simulink model "log_shift_final"  (R2017b)
settings: Solver=FixedStepDiscrete  StartTime=0.0  StopTime=5  RelTol=1e-3
InitFcn:
  | load speech_signal;
  | Fs = 8000;
  | Ts = 1/Fs;
  | 
  | Data_size = 2048;
  | Address_size = log2(Data_size);
  | 
  | FFT_size = 1024
  | FFT_size_half = FFT_size;
  | Frame_shift = 256;
  | Frame_shift_bits = log2(Frame_shift);
  | 
  | Upscale = 32;
libraries: hdlsllib x16, simulink x5, dspxfrm3 x2, dspsigops x1
settings Model: Creator=Ross_admin  LastModifiedBy=s15z586
settings OptimizationCC: BlockReduction=off  ConditionallyExecuteInputs=off  DefaultParameterBehavior=Inlined
settings DebuggingCC: AlgebraicLoopMsg=error  SingleTaskRateTransMsg=error
settings HardwareCC: ProdBitPerPointer=32  ProdBitPerSizeT=32  ProdBitPerPtrDiffT=32  ProdLargestAtomicFloat=None  ProdIntDivRoundTo=Undefined  ProdEndianess=Unspecified  ProdWordSize=32  ProdHWDeviceType=ASIC/FPGA->ASIC/FPGA  TargetBitPerPointer=64  TargetBitPerSizeT=64  TargetBitPerPtrDiffT=64  TargetLongLongMode=on  TargetIntDivRoundTo=Zero  TargetEndianess=LittleEndian  TargetWordSize=64  TargetHWDeviceType=Custom Processor->MATLAB Host Computer  ProdEqTarget=off
settings CodeAppCC: StateflowObjectComments=on

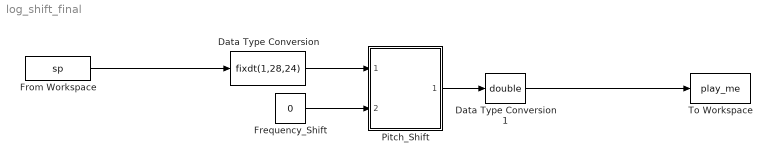
== system log_shift_final ==
  Data Type Conversion : DataTypeConversion  OutDataTypeStr=fixdt(1,28,24)
  Data Type Conversion1 : DataTypeConversion  OutDataTypeStr=double
  Frequency_Shift : Constant  Value=0  OutDataTypeStr=int16  SampleTime=Ts
  From Workspace : FromWorkspace  VariableName=sp  SampleTime=Ts
  Pitch_Shift : Subsystem
  To Workspace : ToWorkspace  VariableName=play_me  SampleTime=-1
  wires:
  Frequency_Shift/1 -> Pitch_Shift/2(Frequency_Shift)
  Pitch_Shift/1(Output) -> Data Type Conversion1/1
  Data Type Conversion/1 -> Pitch_Shift/1(Data_in)
  From Workspace/1 -> Data Type Conversion/1
  Data Type Conversion1/1 -> To Workspace/1

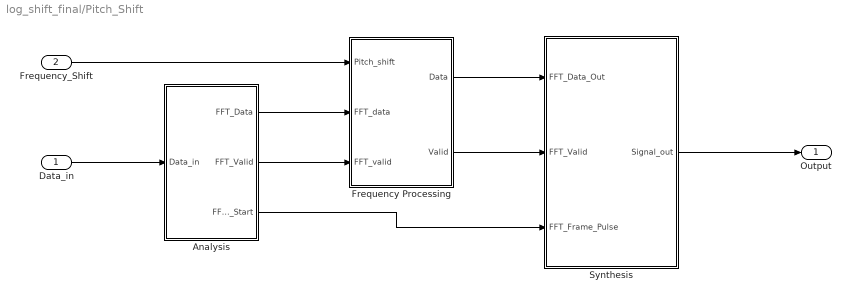
== system log_shift_final/Pitch_Shift ==
  Data_in : Inport
  Frequency_Shift : Inport  Port=2
  Analysis : Subsystem
  Frequency Processing : Subsystem
  Synthesis : Subsystem
  Output : Outport
  wires:
  Data_in/1 -> Analysis/1(Data_in)
  Analysis/3(FFT_Frame_Start) -> Synthesis/3(FFT_Frame_Pulse)
  Synthesis/1(Signal_out) -> Output/1
  Frequency_Shift/1 -> Frequency Processing/1(Pitch_shift)
  Analysis/2(FFT_Valid) -> Frequency Processing/3(FFT_valid)
  Frequency Processing/2(Valid) -> Synthesis/2(FFT_Valid)
  Analysis/1(FFT_Data) -> Frequency Processing/2(FFT_data)
  Frequency Processing/1(Data) -> Synthesis/1(FFT_Data_Out)

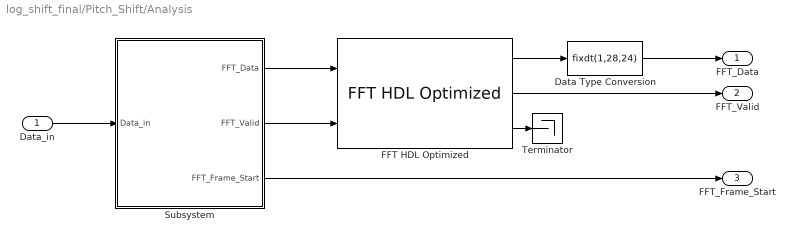
== system log_shift_final/Pitch_Shift/Analysis ==
  Data_in : Inport
  Data Type Conversion : DataTypeConversion  OutDataTypeStr=fixdt(1,28,24)
  FFT HDL Optimized : dspxfrm3/FFT HDL Optimized  FFTLength=1024  Architecture=Burst Radix 2  ComplexMultiplication=Use 4 multipliers and 2 adders  BitReversedOutput=off  BitReversedInput=off  Normalize=on  SimulateUsing=Code generation  RoundingMethod=Floor  ResetInputPort=off  StartOutputPort=off  EndOutputPort=off
      settings: SourceProductName=DSP System Toolbox  SourceProductBaseCode=DS
  Subsystem : Subsystem
  Terminator : Terminator
  FFT_Data : Outport
  FFT_Valid : Outport  Port=2
  FFT_Frame_Start : Outport  Port=3
  wires:
  Data_in/1 -> Subsystem/1(Data_in)
  Subsystem/3(FFT_Frame_Start) -> FFT_Frame_Start/1
  Subsystem/1(FFT_Data) -> FFT HDL Optimized/1
  Subsystem/2(FFT_Valid) -> FFT HDL Optimized/2
  FFT HDL Optimized/2 -> FFT_Valid/1
  FFT HDL Optimized/1 -> Data Type Conversion/1
  Data Type Conversion/1 -> FFT_Data/1
  FFT HDL Optimized/3 -> Terminator/1

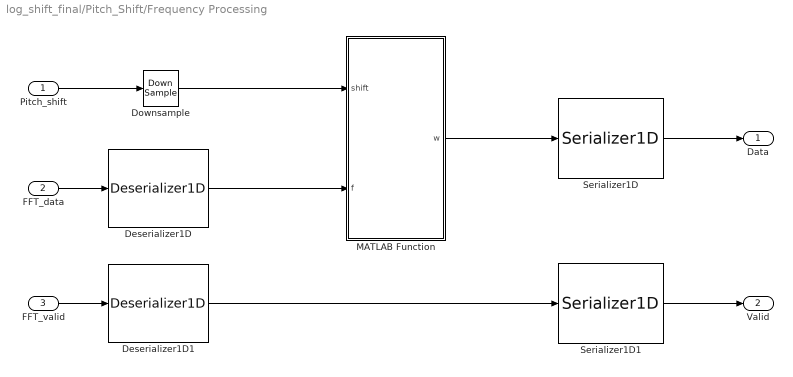
== system log_shift_final/Pitch_Shift/Frequency Processing ==
  Pitch_shift : Inport
  FFT_data : Inport  Port=2
  FFT_valid : Inport  Port=3
  Deserializer1D : hdlsllib/HDL Operations/Deserializer1D  Ratio=1024  IdleCycles=0  InitialCondition=0  startIn=off  validIn=off  validOut=off  inputDataDimensions=-1  inputSampleTime=-1  inputSignalType=auto
      settings: SourceProductName=HDL Coder  SourceProductBaseCode=HD
  Deserializer1D1 : hdlsllib/HDL Operations/Deserializer1D  Ratio=1024  IdleCycles=0  InitialCondition=0  startIn=off  validIn=off  validOut=off  inputDataDimensions=-1  inputSampleTime=-1  inputSignalType=auto
      settings: SourceProductName=HDL Coder  SourceProductBaseCode=HD
  Downsample : DownSample  N=FFT_size/Upscale  RateOptions=Allow multirate processing
  MATLAB Function : MATLAB Function  TreatAsAtomicUnit=on
  Serializer1D : hdlsllib/HDL Operations/Serializer1D  Ratio=1024  IdleCycles=0  validIn=off  startOut=off  validOut=off  inputDataDimensions=-1  inputSampleTime=-1  inputSignalType=auto
      settings: SourceProductName=HDL Coder  SourceProductBaseCode=HD
  Serializer1D1 : hdlsllib/HDL Operations/Serializer1D  Ratio=1024  IdleCycles=0  validIn=off  startOut=off  validOut=off  inputDataDimensions=-1  inputSampleTime=-1  inputSignalType=auto
      settings: SourceProductName=HDL Coder  SourceProductBaseCode=HD
  Data : Outport
  Valid : Outport  Port=2
  wires:
  FFT_valid/1 -> Deserializer1D1/1
  FFT_data/1 -> Deserializer1D/1
  Pitch_shift/1 -> Downsample/1
  Deserializer1D1/1 -> Serializer1D1/1
  Serializer1D1/1 -> Valid/1
  Serializer1D/1 -> Data/1
  Downsample/1 -> MATLAB Function/1(shift)
  Deserializer1D/1 -> MATLAB Function/2(f)
  MATLAB Function/1(w) -> Serializer1D/1

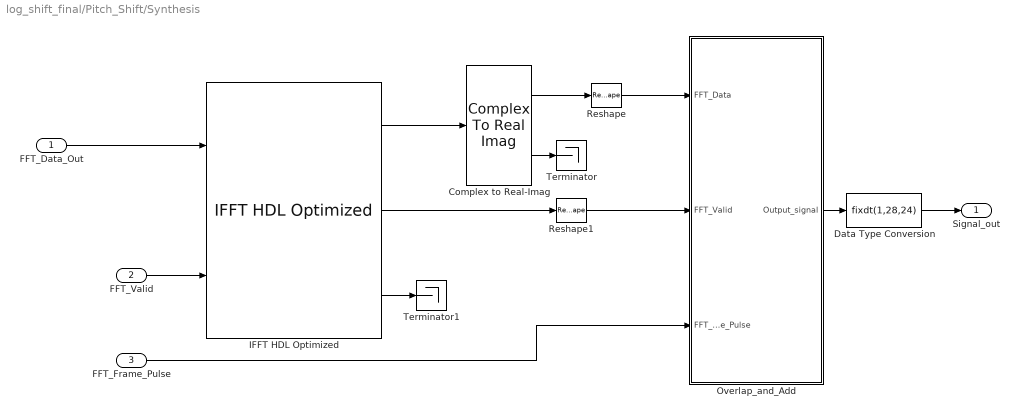
== system log_shift_final/Pitch_Shift/Synthesis ==
  FFT_Data_Out : Inport
  FFT_Valid : Inport  Port=2
  FFT_Frame_Pulse : Inport  Port=3
  Complex to Real-Imag : ComplexToRealImag
  Data Type Conversion : DataTypeConversion  OutDataTypeStr=fixdt(1,28,24)
  IFFT HDL Optimized : dspxfrm3/IFFT HDL Optimized  FFTLength=1024  Architecture=Burst Radix 2  ComplexMultiplication=Use 4 multipliers and 2 adders  BitReversedOutput=off  BitReversedInput=off  Normalize=on  SimulateUsing=Code generation  RoundingMethod=Floor  ResetInputPort=off  StartOutputPort=off  EndOutputPort=off
      settings: SourceProductName=DSP System Toolbox  SourceProductBaseCode=DS
  Overlap_and_Add : Subsystem
  Reshape : Reshape
  Reshape1 : Reshape
  Terminator : Terminator
  Terminator1 : Terminator
  Signal_out : Outport
  wires:
  FFT_Valid/1 -> IFFT HDL Optimized/2
  FFT_Data_Out/1 -> IFFT HDL Optimized/1
  IFFT HDL Optimized/1 -> Complex to Real-Imag/1
  Complex to Real-Imag/2 -> Terminator/1
  Complex to Real-Imag/1 -> Reshape/1
  IFFT HDL Optimized/3 -> Terminator1/1
  IFFT HDL Optimized/2 -> Reshape1/1
  Reshape/1 -> Overlap_and_Add/1(FFT_Data)
  Reshape1/1 -> Overlap_and_Add/2(FFT_Valid)
  FFT_Frame_Pulse/1 -> Overlap_and_Add/3(FFT_Frame_Pulse)
  Overlap_and_Add/1(Output_signal) -> Data Type Conversion/1
  Data Type Conversion/1 -> Signal_out/1

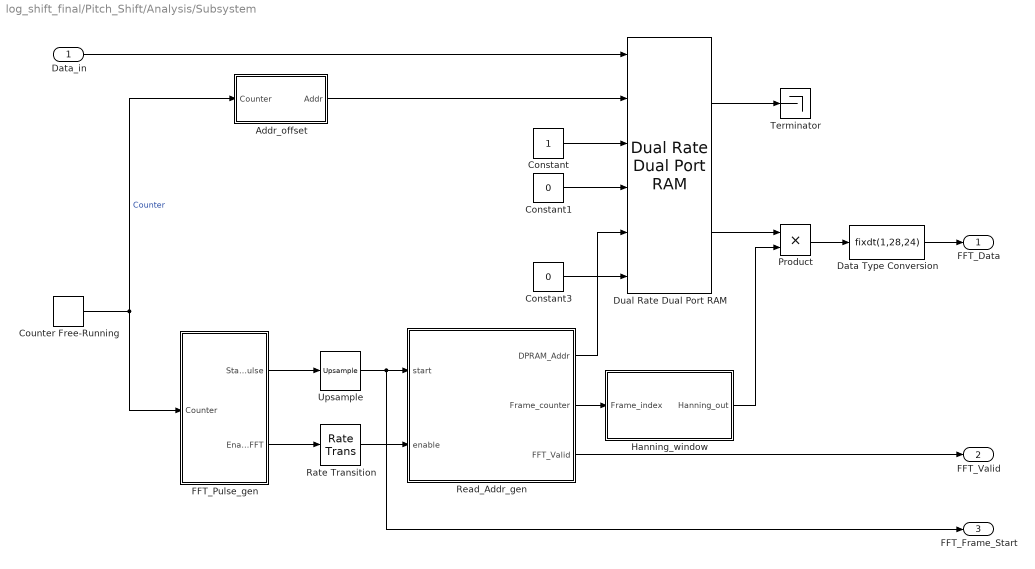
== system log_shift_final/Pitch_Shift/Analysis/Subsystem ==
  Data_in : Inport
  Addr_offset : Subsystem
  Constant : Constant  OutDataTypeStr=boolean  SampleTime=Ts
  Constant1 : Constant  Value=0  OutDataTypeStr=fixdt(1,28,24)  SampleTime=Ts/Upscale
  Constant3 : Constant  Value=0  OutDataTypeStr=boolean  SampleTime=Ts/Upscale
  Counter Free-Running : simulink/Sources/Counter Free-Running  NumBits=Address_size  tsamp=Ts
  Data Type Conversion : DataTypeConversion  OutDataTypeStr=fixdt(1,28,24)
  Dual Rate Dual Port RAM : hdlsllib/HDL RAMs/Dual Rate Dual Port RAM  ram_size=Address_size
      settings: SourceProductName=HDL Coder  SourceProductBaseCode=HD
  FFT_Pulse_gen : Subsystem
  Hanning_window : Subsystem
  Product : Product
  Rate Transition : RateTransition  OutPortSampleTimeOpt=Multiple of input port sample time  OutPortSampleTimeMultiple=1/Upscale  OutPortSampleTime=1/Upscale
  Read_Addr_gen : Subsystem
  Terminator : Terminator
  Upsample : dspsigops/Upsample  N=Upscale  phase=0  RateOptions=Allow multirate processing  ic=0  mode=Unused parameter value
  FFT_Data : Outport
  FFT_Valid : Outport  Port=2
  FFT_Frame_Start : Outport  Port=3
  wires:
  Product/1 -> Data Type Conversion/1
  Dual Rate Dual Port RAM/2 -> Product/1
  Data Type Conversion/1 -> FFT_Data/1
  Hanning_window/1(Hanning_out) -> Product/2
  Read_Addr_gen/2(Frame_counter) -> Hanning_window/1(Frame_index)
  Data_in/1 -> Dual Rate Dual Port RAM/1
  Rate Transition/1 -> Read_Addr_gen/2(enable)
  Read_Addr_gen/1(DPRAM_Addr) -> Dual Rate Dual Port RAM/5
  Counter Free-Running/1 -> Addr_offset/1(Counter), FFT_Pulse_gen/1(Counter)  "Counter"
  FFT_Pulse_gen/2(Enable_FFT) -> Rate Transition/1
  Read_Addr_gen/3(FFT_Valid) -> FFT_Valid/1
  Constant/1 -> Dual Rate Dual Port RAM/3
  Upsample/1 -> FFT_Frame_Start/1, Read_Addr_gen/1(start)
  FFT_Pulse_gen/1(Start_Pulse) -> Upsample/1
  Constant1/1 -> Dual Rate Dual Port RAM/4
  Constant3/1 -> Dual Rate Dual Port RAM/6
  Dual Rate Dual Port RAM/1 -> Terminator/1
  Addr_offset/1(Addr) -> Dual Rate Dual Port RAM/2

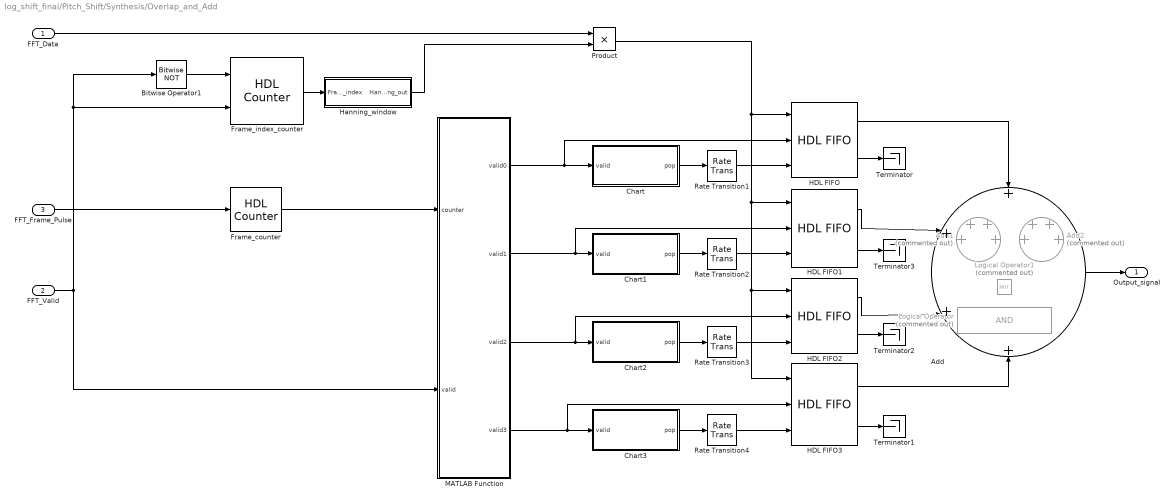
== system log_shift_final/Pitch_Shift/Synthesis/Overlap_and_Add ==
  FFT_Data : Inport
  FFT_Valid : Inport  Port=2
  FFT_Frame_Pulse : Inport  Port=3
  Add : Sum  Inputs=++++
  Add1 : Sum  Commented=on  Inputs=++++
  Add2 : Sum  Commented=on  Inputs=++++
  Bitwise Operator1 : simulink/Logic and Bit Operations/Bitwise Operator  logicop=NOT  UseBitMask=off  BitMask=bin2dec('11011001')  BitMaskRealWorld=Stored Integer
  Chart : Stateflow chart  TreatAsAtomicUnit=on
  Chart1 : Stateflow chart  TreatAsAtomicUnit=on
  Chart2 : Stateflow chart  TreatAsAtomicUnit=on
  Chart3 : Stateflow chart  TreatAsAtomicUnit=on
  Frame_counter : hdlsllib/Sources/HDL Counter  CountType=Free running  CountInit=2  CountStep=1  CountMax=25  CountFromType=Initial value  CountFrom=2  CountResetPort=off  CountLoadPort=off  CountEnbPort=on  CountDirPort=off  CountDataType=Unsigned  CountWordLen=2  CountFracLen=0  CountSampTime=1
      settings: SourceProductBaseCode=HD
  Frame_index_counter : hdlsllib/Sources/HDL Counter  CountType=Count limited  CountInit=0  CountStep=1  CountMax=FFT_size  CountFromType=Initial value  CountFrom=0  CountResetPort=on  CountLoadPort=off  CountEnbPort=on  CountDirPort=off  CountDataType=Unsigned  CountWordLen=Address_size  CountFracLen=0  CountSampTime=1
      settings: SourceProductBaseCode=HD
  HDL FIFO{,1..3} (4 alike) : hdlsllib/HDL RAMs/HDL FIFO  fifo_size=FFT_size  ratio=Upscale  push_msg=Warning  pop_msg=Warning  show_empty=off  show_full=on  show_num=off
      settings: SourceProductName=HDL Coder  SourceProductBaseCode=HD
  Hanning_window : Subsystem
  Logical Operator : Logic  Commented=on  IconShape=distinctive  AllPortsSameDT=off  OutDataTypeStr=boolean
  Logical Operator1 : Logic  Commented=on  Operator=NOT  IconShape=distinctive  AllPortsSameDT=off  OutDataTypeStr=boolean
  MATLAB Function : MATLAB Function  TreatAsAtomicUnit=on
  Product : Product
  Rate Transition{1..4} (4 alike) : RateTransition  OutPortSampleTimeOpt=Multiple of input port sample time  OutPortSampleTimeMultiple=Upscale  OutPortSampleTime=1/Upscale
  Terminator{,1..3} (4 alike) : Terminator
  Output_signal : Outport
  wires:
  Bitwise Operator1/1 -> Frame_index_counter/1
  FFT_Data/1 -> Product/1
  Frame_index_counter/1 -> Hanning_window/1(Frame_index)
  Hanning_window/1(Hanning_out) -> Product/2
  FFT_Valid/1 -> Frame_index_counter/2, Bitwise Operator1/1, MATLAB Function/2(valid)
  HDL FIFO1/1 -> Add/2
  HDL FIFO2/1 -> Add/3
  HDL FIFO3/1 -> Add/4
  HDL FIFO/1 -> Add/1
  Frame_counter/1 -> MATLAB Function/1(counter)
  MATLAB Function/1(valid0) -> HDL FIFO/2, Chart/1(valid)
  MATLAB Function/2(valid1) -> HDL FIFO1/2, Chart1/1(valid)
  MATLAB Function/3(valid2) -> HDL FIFO2/2, Chart2/1(valid)
  MATLAB Function/4(valid3) -> HDL FIFO3/2, Chart3/1(valid)
  Product/1 -> HDL FIFO2/1, HDL FIFO3/1, HDL FIFO1/1, HDL FIFO/1
  Add/1 -> Output_signal/1
  Chart1/1(pop) -> Rate Transition2/1
  Chart2/1(pop) -> Rate Transition3/1
  Chart3/1(pop) -> Rate Transition4/1
  Chart/1(pop) -> Rate Transition1/1
  Rate Transition1/1 -> HDL FIFO/3
  Rate Transition2/1 -> HDL FIFO1/3
  Rate Transition3/1 -> HDL FIFO2/3
  Rate Transition4/1 -> HDL FIFO3/3
  FFT_Frame_Pulse/1 -> Frame_counter/1
  HDL FIFO/2 -> Terminator/1
  HDL FIFO2/2 -> Terminator2/1
  HDL FIFO1/2 -> Terminator3/1
  HDL FIFO3/2 -> Terminator1/1

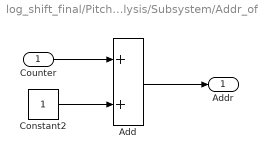
== system log_shift_final/Pitch_Shift/Analysis/Subsystem/Addr_offset ==
  Counter : Inport
  Add : Sum  AccumDataTypeStr=fixdt(0,Address_size,0)
  Constant2 : Constant  OutDataTypeStr=fixdt(0,Address_size,0)  SampleTime=Ts
  Addr : Outport
  wires:
  Add/1 -> Addr/1
  Counter/1 -> Add/1
  Constant2/1 -> Add/2

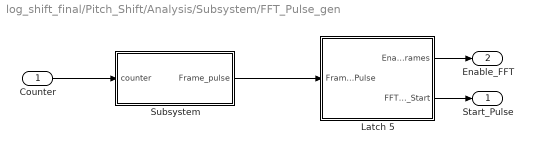
== system log_shift_final/Pitch_Shift/Analysis/Subsystem/FFT_Pulse_gen ==
  Counter : Inport
  "Latch 5 " : Subsystem
  Subsystem : Subsystem
  Start_Pulse : Outport
  Enable_FFT : Outport  Port=2
  wires:
  Counter/1 -> Subsystem/1("counter ")
  Subsystem/1(Frame_pulse) -> "Latch 5 "/1(Frame_Pulse)
  "Latch 5 "/2(FFT_Frame_Start) -> Start_Pulse/1
  "Latch 5 "/1(Enable_FFT_Frames) -> Enable_FFT/1

== system log_shift_final/Pitch_Shift/Analysis/Subsystem/Hanning_window ==
  Frame_index : Inport
  1-D Lookup Table : Lookup_n-D  NumberOfTableDimensions=1  LookupTableObject=''  BreakpointsForDimension1=[0:FFT_size]  BreakpointsForDimension1FirstPoint=10  BreakpointsForDimension2FirstPoint=10  BreakpointsForDimension1Spacing=12  BreakpointsForDimension2Spacing=12  IndexSearchMethod=Evenly spaced points  Table=hanning(FFT_size+1)  InterpMethod=Flat  DiagnosticForOutOfRangeInput=Error  OutDataTypeStr=fixdt(1,16,14)  RndMeth=Simplest  InputSameDT=on
  Unit Delay : UnitDelay  SampleTime=-1
  Hanning_out : Outport
  wires:
  1-D Lookup Table/1 -> Unit Delay/1
  Unit Delay/1 -> Hanning_out/1
  Frame_index/1 -> 1-D Lookup Table/1

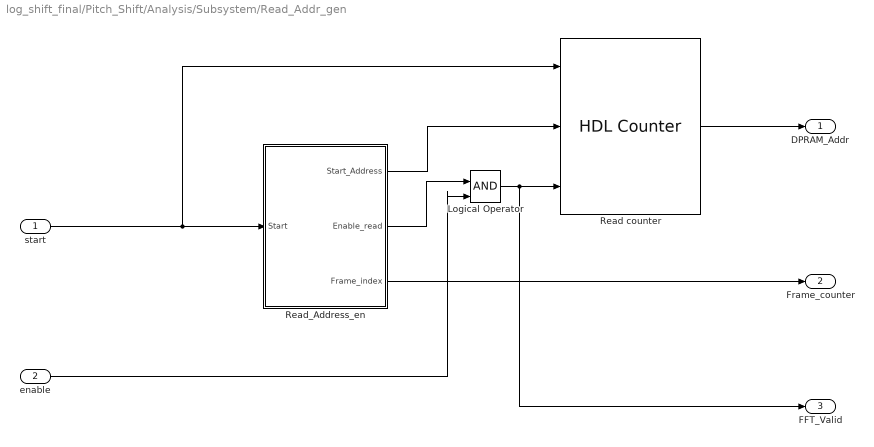
== system log_shift_final/Pitch_Shift/Analysis/Subsystem/Read_Addr_gen ==
  start : Inport
  enable : Inport  Port=2
  Logical Operator : Logic  IconShape=distinctive  AllPortsSameDT=off  OutDataTypeStr=boolean
  Read counter : hdlsllib/Sources/HDL Counter  CountType=Free running  CountInit=Data_size - 10  CountStep=1  CountMax=Data_size  CountFromType=Specify  CountFrom=0  CountResetPort=off  CountLoadPort=on  CountEnbPort=on  CountDirPort=off  CountDataType=Unsigned  CountWordLen=Address_size  CountFracLen=0  CountSampTime=1
      settings: SourceProductBaseCode=HD
  Read_Address_en : Subsystem
  DPRAM_Addr : Outport
  Frame_counter : Outport  Port=2
  FFT_Valid : Outport  Port=3
  wires:
  start/1 -> Read counter/1, Read_Address_en/1(Start)
  Read counter/1 -> DPRAM_Addr/1
  Read_Address_en/3(Frame_index) -> Frame_counter/1
  Read_Address_en/2(Enable_read) -> Logical Operator/1
  enable/1 -> Logical Operator/2
  Logical Operator/1 -> FFT_Valid/1, Read counter/3
  Read_Address_en/1(Start_Address) -> Read counter/2

== system log_shift_final/Pitch_Shift/Synthesis/Overlap_and_Add/Hanning_window ==
  Frame_index : Inport
  1-D Lookup Table : Lookup_n-D  NumberOfTableDimensions=1  LookupTableObject=''  BreakpointsForDimension1=[0:FFT_size]  BreakpointsForDimension1FirstPoint=10  BreakpointsForDimension2FirstPoint=10  BreakpointsForDimension1Spacing=12  BreakpointsForDimension2Spacing=12  IndexSearchMethod=Evenly spaced points  Table=hanning(FFT_size+1)  InterpMethod=Flat  DiagnosticForOutOfRangeInput=Error  OutDataTypeStr=fixdt(1,16,14)  RndMeth=Simplest  InputSameDT=on
  Unit Delay : UnitDelay  SampleTime=-1
  Hanning_out : Outport
  wires:
  1-D Lookup Table/1 -> Unit Delay/1
  Unit Delay/1 -> Hanning_out/1
  Frame_index/1 -> 1-D Lookup Table/1

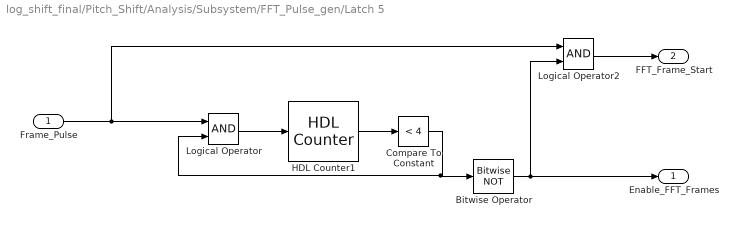
== system log_shift_final/Pitch_Shift/Analysis/Subsystem/FFT_Pulse_gen/Latch 5  ==
  Frame_Pulse : Inport
  Bitwise Operator : simulink/Logic and Bit Operations/Bitwise Operator  logicop=NOT  UseBitMask=off  BitMask=bin2dec('11011001')  BitMaskRealWorld=Stored Integer
  Compare To Constant : simulink/Logic and Bit Operations/Compare To Constant  relop=<  const=4  OutDataTypeStr=boolean
  HDL Counter1 : hdlsllib/Sources/HDL Counter  CountType=Count limited  CountInit=0  CountStep=1  CountMax=4  CountFromType=Initial value  CountFrom=0  CountResetPort=off  CountLoadPort=off  CountEnbPort=on  CountDirPort=off  CountDataType=Unsigned  CountWordLen=5  CountFracLen=0  CountSampTime=1
      settings: SourceProductBaseCode=HD
  Logical Operator : Logic  AllPortsSameDT=off  OutDataTypeStr=boolean
  Logical Operator2 : Logic  AllPortsSameDT=off  OutDataTypeStr=boolean
  Enable_FFT_Frames : Outport
  FFT_Frame_Start : Outport  Port=2
  wires:
  Frame_Pulse/1 -> Logical Operator2/1, Logical Operator/1
  Logical Operator/1 -> HDL Counter1/1
  HDL Counter1/1 -> Compare To Constant/1
  Compare To Constant/1 -> Bitwise Operator/1, Logical Operator/2
  Bitwise Operator/1 -> Enable_FFT_Frames/1, Logical Operator2/2
  Logical Operator2/1 -> FFT_Frame_Start/1

== system log_shift_final/Pitch_Shift/Analysis/Subsystem/FFT_Pulse_gen/Subsystem ==
  "counter " : Inport
  Bit Slice : hdlsllib/Logic and Bit Operations/Bit Slice  lidx=7  ridx=0
  Compare To Zero : simulink/Logic and Bit Operations/Compare To Zero  relop===  OutDataTypeStr=boolean
  Frame_pulse : Outport
  wires:
  "counter "/1 -> Bit Slice/1
  Bit Slice/1 -> Compare To Zero/1
  Compare To Zero/1 -> Frame_pulse/1

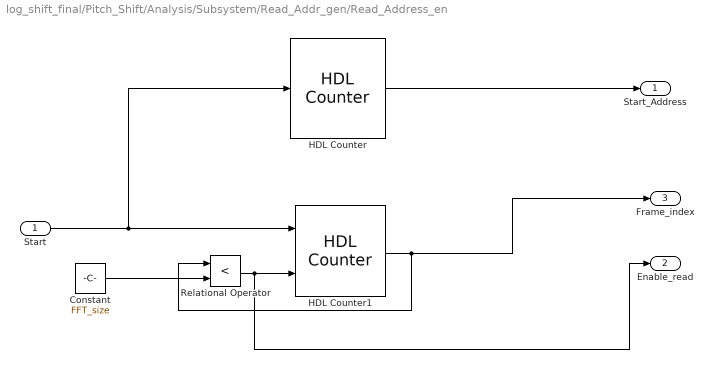
== system log_shift_final/Pitch_Shift/Analysis/Subsystem/Read_Addr_gen/Read_Address_en ==
  Start : Inport
  Constant : Constant  Value=FFT_size  OutDataTypeStr=fixdt(1,11)  SampleTime=Ts/Upscale
  HDL Counter : hdlsllib/Sources/HDL Counter  CountType=Free running  CountInit=0  CountStep=Frame_shift  CountMax=1024  CountFromType=Specify  CountFrom=0  CountResetPort=off  CountLoadPort=off  CountEnbPort=on  CountDirPort=off  CountDataType=Unsigned  CountWordLen=Address_size  CountFracLen=0  CountSampTime=1
      settings: SourceProductBaseCode=HD
  HDL Counter1 : hdlsllib/Sources/HDL Counter  CountType=Count limited  CountInit=0  CountStep=1  CountMax=FFT_size  CountFromType=Specify  CountFrom=0  CountResetPort=on  CountLoadPort=off  CountEnbPort=on  CountDirPort=off  CountDataType=Unsigned  CountWordLen=Address_size  CountFracLen=0  CountSampTime=1
      settings: SourceProductBaseCode=HD
  Relational Operator : RelationalOperator  Operator=<  OutDataTypeStr=boolean  RndMeth=Nearest
  Start_Address : Outport
  Enable_read : Outport  Port=2
  Frame_index : Outport  Port=3
  wires:
  Start/1 -> HDL Counter/1, HDL Counter1/1
  Relational Operator/1 -> Enable_read/1, HDL Counter1/2
  HDL Counter1/1 -> Relational Operator/1, Frame_index/1
  HDL Counter/1 -> Start_Address/1
  Constant/1 -> Relational Operator/2

== stateflow chart log_shift_final/Pitch_Shift/Synthesis/Overlap_and_Add/Chart1 ==
  settings: executeAtInitialization=1
  state Start
    entry:pop = fi(0, 0, 1, 0)
  state valid_low
    entry:pop = fi(0, 0, 1, 0)
  state valid_high
    entry:pop = fi(0, 0, 1, 0)
  state Done
    entry:pop = fi(1, 0, 1, 0)
  (default) -> Start
  Start -> valid_low : [valid==0]
  valid_low -> valid_high [order 2] : [valid == 1]
  valid_high -> Done [order 1] : [valid == 0]
  valid_low -> valid_low [order 1] : [valid == 0]
  valid_high -> valid_high [order 2] : [valid == 1]
  data: valid input; pop output

== stateflow chart log_shift_final/Pitch_Shift/Synthesis/Overlap_and_Add/Chart2 ==
  settings: executeAtInitialization=1
  state Start
    entry:pop = fi(0, 0, 1, 0)
  state valid_low
    entry:pop = fi(0, 0, 1, 0)
  state valid_high
    entry:pop = fi(0, 0, 1, 0)
  state Done
    entry:pop = fi(1, 0, 1, 0)
  (default) -> Start
  Start -> valid_low : [valid==0]
  valid_low -> valid_high [order 2] : [valid == 1]
  valid_high -> Done [order 1] : [valid == 0]
  valid_low -> valid_low [order 1] : [valid == 0]
  valid_high -> valid_high [order 2] : [valid == 1]
  data: valid input; pop output

== stateflow chart log_shift_final/Pitch_Shift/Synthesis/Overlap_and_Add/Chart ==
  settings: executeAtInitialization=1
  state Start
    entry:pop = fi(0, 0, 1, 0);
  state valid_low
    entry:pop = fi(0, 0, 1, 0);
  state valid_high
    entry:pop = fi(0, 0, 1, 0);
  state Done
    entry:pop = fi(1, 0, 1, 0);
  (default) -> Start
  Start -> valid_low : [valid==0]
  valid_low -> valid_high [order 2] : [valid == 1]
  valid_high -> Done [order 1] : [valid == 0]
  valid_low -> valid_low [order 1] : [valid == 0]
  valid_high -> valid_high [order 2] : [valid == 1]
  data: valid input; pop output

== stateflow chart log_shift_final/Pitch_Shift/Synthesis/Overlap_and_Add/Chart3 ==
  settings: executeAtInitialization=1
  state Start
    entry:pop = fi(0, 0, 1, 0)
  state valid_low
    entry:pop = fi(0, 0, 1, 0)
  state valid_high
    entry:pop = fi(0, 0, 1, 0)
  state Done
    entry:pop = fi(1, 0, 1, 0)
  (default) -> Start
  Start -> valid_low : [valid==0]
  valid_low -> valid_high [order 2] : [valid == 1]
  valid_high -> Done [order 1] : [valid == 0]
  valid_low -> valid_low [order 1] : [valid == 0]
  valid_high -> valid_high [order 2] : [valid == 1]
  data: valid input; pop output

== matlab function log_shift_final/Pitch_Shift/Synthesis/Overlap_and_Add/MATLAB Function ==
  data: counter input; valid0 output; valid1 output; valid2 output; valid3 output; valid input
function [valid0, valid1, valid2, valid3]= fcn(counter, valid)
switch(counter)
    case 0
        valid0 = valid;
        valid1 = false;
        valid2 = false;
        valid3 = false;
    case 1
        valid0 = false;
        valid1 = valid;
        valid2 = false;
        valid3 = false;
    case 2
        valid0 = false;
        valid1 = false;
        valid2 = valid;
        valid3 = false;
    case 3
        valid0 = false;
        valid1 = false;
        valid2 = false;
        valid3 = valid;
    otherwise
        valid0 = false;
        valid1 = false;
        valid2 = false;
        valid3 = false;
end

== matlab function log_shift_final/Pitch_Shift/Frequency Processing/MATLAB Function ==
  data: shift input; f input; w output
function w = fcn(shift,f)

if shift > 0
    logshift = floor(log(double(shift)));
else
    logshift = -1*floor(log(double(abs(shift))));
end

N = length(f);
Nd2 = N/2;
w = fi(complex(zeros(N,1)), 1, 28, 24);

if shift == 0
    w = f;
else
    w(1)     = fi(complex(0), 1 , 28, 24);
    w(Nd2+1) = fi(complex(0), 1 , 28, 24);
    
    if shift > 0  % increase the frequencies
        for i=2:Nd2
            if i <= shift
                w(i) = fi(complex(0), 1 , 28, 24); % fill in vacated positive frequencies with zeros
            else
                w(i) = f(i-logshift);
            end
        end
        for i=N:-1:Nd2+2
            if i > N-shift
                w(i) = fi(complex(0), 1 , 28, 24);
            else
                w(i) = f(i+logshift);
            end
        end
    end
    
    if shift < 0  % decrease the frequencies
        
        for i=Nd2:-1:2
            if i > Nd2 + shift
                w(i) = fi(complex(0), 1 , 28, 24);
            else
                w(i) = f(i-logshift);
            end
        end
        
        for i=Nd2+2:N
            if i <= Nd2 + 2 - shift
                w(i) = fi(complex(0), 1 , 28, 24);
            else
                w(i) = f(i+logshift);
            end
        end
    end
end
end
